simulink model "test_aw"  (Simulink 4.00)
settings: Solver=FixedStepDiscrete  StartTime=0.0  StopTime=60  FixedStep=0.05  RelTol=1e-3
undefined symbols (not defined in the file or in its folder): motor_1
libraries: rst_controller_lib x3
settings Model: LastModifiedBy=bsaunder

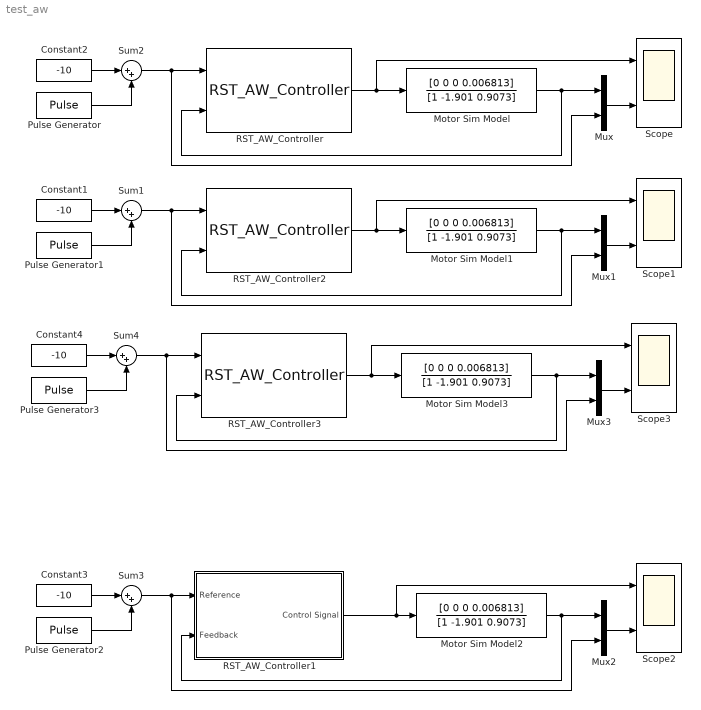
== system test_aw ==
  Constant{1..4} (4 alike) : Constant  Value=-10
  Motor Sim Model{,1..3} (4 alike) : DiscreteFilter  Numerator=[0 0 0 0.006813]  Denominator=[1 -1.901 0.9073]  SampleTime=0.05  Realization=auto
      settings: RTWStateStorageClass=Auto
  Mux{,1..3} (4 alike) : Mux  Inputs=2
  Pulse Generator{,1..3} (4 alike) : DiscretePulseGenerator  PulseType=Time-based  Amplitude=20  Period=20  PulseWidth=50  PhaseDelay=0  SampleTime=1
  RST_AW_Controller : rst_controller_lib/RST_AW_Controller  Get_Controller_file=on  controll_fname='GLA_BEN_04_01_12_motor_1'  R=motor_1.Controller_Design_1.rst_ctrl.R  S=motor_1.Controller_Design_1.rst_ctrl.S  T=motor_1.Controller_Design_1.rst_ctrl.T  Aaw=motor_1.Controller_Design_1.rst_ctrl.Aaw  Aaw_R=motor_1.Controller_Design_1.rst_ctrl.Aaw_R  out_limit=[0 100]  sT=0.05
  RST_AW_Controller1 : Subsystem  mask(RST Controller Design){Get_Controller_file=on, controll_fname='GLA_BEN_04_01_12_motor_3', R=motor_1.Controller_Design_1.rst_ctrl.R, S=motor_1.Controller_Design_1.rst_ctrl.S, T=motor_1.Controller_Design_1.rst_ctrl.T, Aaw=motor_1.Controller_Design_1.rst_ctrl.Aaw, Aaw_R=motor_1.Controller_Design_1.rst_ctrl.Aaw_R, out_limit=[0 100], sT=0.05}
      mask prompts: Get_Controller_file "Get Controller from File"; controll_fname "Controller file name"; Aaw_R "Aaw - R"; out_limit "Output limitations"; sT "Sample time"
      mask help: Design of a controller that takes the form R*u = T*ref - S*output
      mask init:
      | if Get_Controller_file
      |    ctr_data = load(['Controllers\', controll_fname]);
      |    R = ctr_data.controllerData.rst.rst_ctrl.R;
      |    S = ctr_data.controllerData.rst.rst_ctrl.S;
      |    T = ctr_data.controllerData.rst.rst_ctrl.T;
      |    Aaw = ctr_data.controllerData.rst.rst_ctrl.Aaw;
      |    Aaw_R = ctr_data.controllerData.rst.rst_ctrl.Aaw_R;
      | end
      settings: RTWFcnNameOpts=Auto  RTWFileNameOpts=Auto
      mask CallbackString:
      | mv = get_param(gcb, 'MaskValues');
      |  if strcmp(mv{1}, 'on') a = 'on'; b = 'off';
      |  else a = 'off'; b = 'on';
      |  end;
      |  me = get_param(gcb, 'MaskEnables');
      |  me{2} = a;
      |  me{3} = b;
      |  me{4} = b;
      |  me{5} = b;
      |  me{6} = b;
      |  me{7} = b;
      |  set_param(gcb, 'MaskEnables', me);
      | ||||||||
      mask Display:
      | port_label('input', 1, 'Ref');
      | port_label('input', 2, 'Feedbk');
      | 
      | plot([0.01 0.05 0.01].*0.6+0.3, [0.82 0.8 0.78]);
      | plot([0.95 0.99 0.95].*0.6+0.3, [0.82 0.8 0.78]);
      | plot([0.52 0.48 0.52].*0.6+0.3, [0.22 0.2 0.18]);
      | 
      | plot([0.05 0.15 0.25; 0.25 0.15 0.35].*0.6+0.3, [0.8 0.2 0.6; 0.8 0.8 0.3]);
      | plot((0.25+0.1.*sin([0:pi/90:pi])).*0.6+0.3,0.7+0.1.*cos([0:pi/90:pi]));
      | plot([0.18 0.18; 0.18 0.25].*0.6+0.3, [0.3 0.75; 0.75 0.75]);
      | 
      | plot([0.35 0.5; 0.5 0.99].*0.6+0.3, [0.3 0.8; 0.3 0.8]);
      | plot((0.5+0.1.*sin([-pi:pi/90:0])).*0.6+0.3,0.7+0.1.*cos([0:pi/90:pi]));
      | plot((0.5+0.1.*sin([0:pi/90:pi])).*0.6+0.3,0.45+0.15.*cos([0:pi/90:pi]));
      | plot((0.5+0.07.*sin([-pi:pi/90:0])).*0.6+0.3,0.7+0.05.*cos([0:pi/90:pi]));
      | plot([0.5 0.6].*0.6+0.3, [0.75 0.75]);
      | 
      | plot([0.75 0.75; 0.75 0.15].*0.6+0.3, [0.8 0.2; 0.2 0.2]);
      | plot([0.85 0.78; 0.78 0.78].*0.6+0.3, [0.75 0.75; 0.75 0.3]);
      | 
      | text(0.5, 0.1, 'Anti-reset Control', 'VerticalAlignment', 'middle', 'HorizontalAlignment', 'center');
  RST_AW_Controller2 : rst_controller_lib/RST_AW_Controller  Get_Controller_file=on  controll_fname='GLA_BEN_04_01_12_motor_2'  R=motor_1.Controller_Design_1.rst_ctrl.R  S=motor_1.Controller_Design_1.rst_ctrl.S  T=motor_1.Controller_Design_1.rst_ctrl.T  Aaw=motor_1.Controller_Design_1.rst_ctrl.Aaw  Aaw_R=motor_1.Controller_Design_1.rst_ctrl.Aaw_R  out_limit=[0 100]  sT=0.05
  RST_AW_Controller3 : rst_controller_lib/RST_AW_Controller  Get_Controller_file=on  controll_fname='GLA_BEN_04_01_12_motor_3'  R=motor_1.Controller_Design_1.rst_ctrl.R  S=motor_1.Controller_Design_1.rst_ctrl.S  T=motor_1.Controller_Design_1.rst_ctrl.T  Aaw=motor_1.Controller_Design_1.rst_ctrl.Aaw  Aaw_R=motor_1.Controller_Design_1.rst_ctrl.Aaw_R  out_limit=[0 100]  sT=0.05
  Scope{,1..3} (4 alike) : Scope  NumInputPorts=2
      Scope settings: TimeRange=60  YMin=15~0  YMax=65~80  SaveToWorkspace=off  SaveName=ScopeData  LimitDataPoints=on  MaxDataPoints=5000
      Scope1 settings: TimeRange=60  YMin=15~0  YMax=65~80  SaveToWorkspace=off  LimitDataPoints=on  MaxDataPoints=5000
      Scope2 settings: TimeRange=60  YMin=15~0  YMax=65~80  SaveToWorkspace=off  SaveName=ScopeData2  LimitDataPoints=on  MaxDataPoints=5000
      Scope3 settings: TimeRange=60  YMin=15~0  YMax=65~80  SaveToWorkspace=off  SaveName=ScopeData6  LimitDataPoints=on  MaxDataPoints=5000
  Sum{1..4} (4 alike) : Sum  Inputs=|++  SaturateOnIntegerOverflow=on
  wires:
  Sum2/1 -> Mux/2, RST_AW_Controller/1
  Constant2/1 -> Sum2/1
  Pulse Generator/1 -> Sum2/2
  RST_AW_Controller/1 -> Scope/1, Motor Sim Model/1
  Motor Sim Model/1 -> Mux/1, RST_AW_Controller/2
  Mux/1 -> Scope/2
  Sum3/1 -> Mux2/2, RST_AW_Controller1/1(Reference)
  Constant3/1 -> Sum3/1
  Pulse Generator2/1 -> Sum3/2
  RST_AW_Controller1/1(Control Signal) -> Scope2/1, Motor Sim Model2/1
  Motor Sim Model2/1 -> Mux2/1, RST_AW_Controller1/2(Feedback)
  Mux2/1 -> Scope2/2
  Sum1/1 -> RST_AW_Controller2/1, Mux1/2
  Constant1/1 -> Sum1/1
  Pulse Generator1/1 -> Sum1/2
  RST_AW_Controller2/1 -> Motor Sim Model1/1, Scope1/1
  Motor Sim Model1/1 -> RST_AW_Controller2/2, Mux1/1
  Mux1/1 -> Scope1/2
  Sum4/1 -> Mux3/2, RST_AW_Controller3/1
  Constant4/1 -> Sum4/1
  Pulse Generator3/1 -> Sum4/2
  RST_AW_Controller3/1 -> Scope3/1, Motor Sim Model3/1
  Motor Sim Model3/1 -> Mux3/1, RST_AW_Controller3/2
  Mux3/1 -> Scope3/2

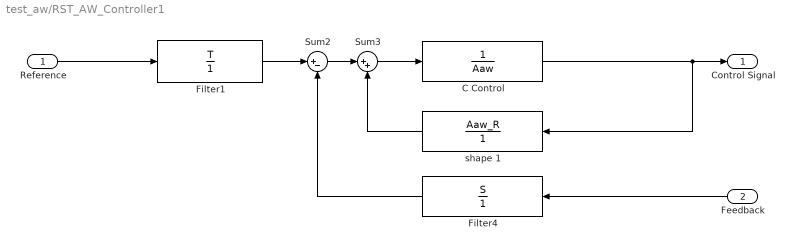
== system test_aw/RST_AW_Controller1 ==
  Reference : Inport  Port=1  LatchInput=off
  Feedback : Inport  Orientation=left  Port=2  LatchInput=off
  C Control : DiscreteFilter  Numerator=1  Denominator=Aaw  SampleTime=sT  Realization=auto
      settings: RTWStateStorageClass=Auto
  Filter1 : DiscreteFilter  Numerator=T  Denominator=1  SampleTime=sT  Realization=auto
      settings: RTWStateStorageClass=Auto
  Filter4 : DiscreteFilter  Orientation=left  Numerator=S  Denominator=1  SampleTime=sT  Realization=auto
      settings: RTWStateStorageClass=Auto
  Sum2 : Sum  Inputs=|+-  SaturateOnIntegerOverflow=on
  Sum3 : Sum  Inputs=|++  SaturateOnIntegerOverflow=on
  shape 1 : DiscreteFilter  Orientation=left  Numerator=Aaw_R  Denominator=1  SampleTime=sT  Realization=auto
      settings: RTWStateStorageClass=Auto
  Control Signal : Outport  Port=1
  wires:
  Filter4/1 -> Sum2/2
  Sum2/1 -> Sum3/1
  Filter1/1 -> Sum2/1
  Feedback/1 -> Filter4/1
  shape 1/1 -> Sum3/2
  C Control/1 -> Control Signal/1, shape 1/1
  Sum3/1 -> C Control/1
  Reference/1 -> Filter1/1
